simulink model "gm_pwm_fpga_slrt"  (R2020b)
settings: Solver=FixedStepDiscrete  StartTime=0.0  StopTime=5  FixedStep=1e-3  RelTol=1e-3
PostLoadFcn:
  | try
  | cell = struct2cell(dir(fullfile(speedgoatroot_hdlb, 'hdlsrc', 'pwm', '*.vhd')));
  | addSourceFiles = strjoin(fullfile(cell(2,:),cell(1,:)), ';');
  | hdlset_param('pwm_example_hdlc/DUT PWM and CAP', 'IPCoreAdditionalFiles', addSourceFiles);
  | end
undefined symbols (not defined in the file): IO334
libraries: speedgoatlib_hdlCoder_IO3xx x5, pwm_cpulib x1
settings Model: ModifiedByFormat=Speedgoat GmbH  Creator=Speedgoat GmbH  LastModifiedBy=Speedgoat GmbH
settings SolverCC: ConcurrentTasks=on  PositivePriorityOrder=on
settings DataIOCC: LimitDataPoints=on  SaveFormat=Array  ReturnWorkspaceOutputs=off
settings OptimizationCC: BlockReduction=off  ConditionallyExecuteInputs=off  DefaultParameterBehavior=Inlined  OptimizeBlockIOStorage=off
settings DebuggingCC: AlgebraicLoopMsg=error  UnderspecifiedInitializationDetection=Classic  MergeDetectMultiDrivingBlocksExec=none  SolverPrmCheckMsg=warning  SingleTaskRateTransMsg=error  TasksWithSamePriorityMsg=none  PregeneratedLibrarySubsystemCodeDiagnostic=none  SFUnexpectedBacktrackingDiag=warning  SFNoUnconditionalDefaultTransitionDiag=warning  SFExecutionAtInitializationDiag=none  ArithmeticOperatorsInVariantConditions=warning
settings HardwareCC: ProdBitPerLong=64  ProdLongLongMode=on  ProdHWDeviceType=Intel->x86-64 (Linux 64)
settings ModelReferenceCC: PropagateSignalLabelsOutOfModel=off
settings SFSimCC: SimUseLocalCustomCode=off  CustomCodeUndefinedFunction=UseInterfaceOnly
settings RTWCC: Description=Simulink Real-Time  SystemTargetFile=slrealtime.tlc  TemplateMakefile=slrealtime_default_tmf  RTWUseLocalCustomCode=off  Toolchain=Simulink Real-Time Toolchain  BuildConfiguration=Faster Runs  CodeExecutionProfiling=on  TargetLang=C++
settings CodeAppCC: StateflowObjectComments=on
settings ConfigComp: CovMetricSettings=dw  CovSaveCumulativeToWorkspaceVar=on  CovSaveSingleToWorkspaceVar=on  CovExternalEMLEnable=off

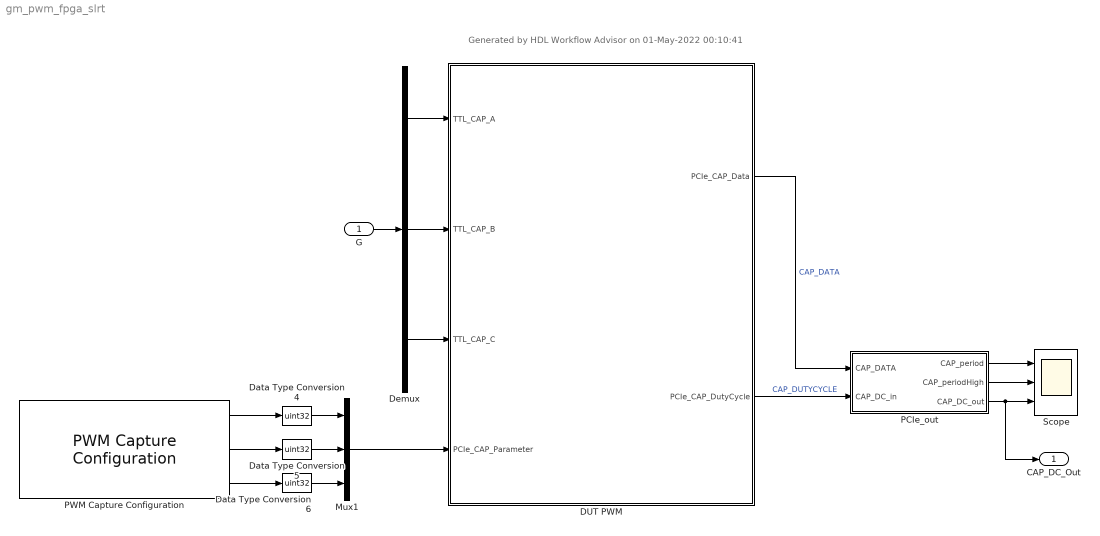
== system gm_pwm_fpga_slrt ==
  note: Generated by HDL Workflow Advisor on 01-May-2022 00:10:41
  G : Inport
  DUT PWM : Subsystem  mask(Speedgoat IO334-325k Interface Block){module_id=1, slot=-1, ts=-1, PullRPort0=pull-up 3.3V, VioPort0=3.3V, PullRPort1=pull-up 3.3V, VioPort1=3.3V, PullRPort2=pull-up 3.3V, VioPort2=3.3V, PullRPort3=pull-up 3.3V, VioPort3=3.3V, PullRPort4=pull-up 3.3V, VioPort4=3.3V, PullRPort5=pull-up 3.3V, VioPort5=3.3V, PullRPort6=pull-up 3.3V, VioPort6=3.3V, FpgaFreq=100}
      mask prompts: module_id "FPGA Module Identifier:"; slot "PCI slot (-1: autosearch):"; ts "Sample time:"; PullRPort0 "pull resistor"; VioPort0 "I/O voltage"; PullRPort1 "pull resistor"; VioPort1 "I/O voltage"; PullRPort2 "pull resistor"; VioPort2 "I/O voltage"; PullRPort3 "pull resistor"; VioPort3 "I/O voltage"; PullRPort4 "pull resistor"; VioPort4 "I/O voltage"; PullRPort5 "pull resistor"; VioPort5 "I/O voltage"; PullRPort6 "pull resistor"; VioPort6 "I/O voltage"; FpgaFreq "FPGA Frequency [MHz]"
      mask help: Simulink Real-Time Interface Block for Speedgoat IO334-325k.
      mask init:
      | hdlslrt.backend.mfpgaparameters;
      mask Help: eval('speedgoatdoc_hdlc')
      mask TypeOptions PullRPort0: Port Settings -2x/PullRPort0
      mask Callback PullRPort0: sg_fpga_HDLCoder_io3xx_2x_m(2)
      mask TypeOptions VioPort0: Port Settings -2x/VioPort0
      mask Callback VioPort0: sg_fpga_HDLCoder_io3xx_2x_m(2)
      mask TypeOptions PullRPort1: Port Settings -2x/PullRPort1
      mask Callback PullRPort1: sg_fpga_HDLCoder_io3xx_2x_m(2)
      mask TypeOptions VioPort1: Port Settings -2x/VioPort1
      mask Callback VioPort1: sg_fpga_HDLCoder_io3xx_2x_m(2)
      mask TypeOptions PullRPort2: Port Settings -2x/PullRPort2
      mask Callback PullRPort2: sg_fpga_HDLCoder_io3xx_2x_m(2)
      mask TypeOptions VioPort2: Port Settings -2x/VioPort2
      mask Callback VioPort2: sg_fpga_HDLCoder_io3xx_2x_m(2)
      mask TypeOptions PullRPort3: Port Settings -2x/PullRPort3
      mask Callback PullRPort3: sg_fpga_HDLCoder_io3xx_2x_m(2)
      mask TypeOptions VioPort3: Port Settings -2x/VioPort3
      mask Callback VioPort3: sg_fpga_HDLCoder_io3xx_2x_m(2)
      mask TypeOptions PullRPort4: Port Settings -2x/PullRPort4
      mask Callback PullRPort4: sg_fpga_HDLCoder_io3xx_2x_m(2)
      mask TypeOptions VioPort4: Port Settings -2x/VioPort4
      mask Callback VioPort4: sg_fpga_HDLCoder_io3xx_2x_m(2)
      mask TypeOptions PullRPort5: Port Settings -2x/PullRPort5
      mask Callback PullRPort5: sg_fpga_HDLCoder_io3xx_2x_m(2)
      mask TypeOptions VioPort5: Port Settings -2x/VioPort5
      mask Callback VioPort5: sg_fpga_HDLCoder_io3xx_2x_m(2)
      mask TypeOptions PullRPort6: Port Settings -2x/PullRPort6
      mask Callback PullRPort6: sg_fpga_HDLCoder_io3xx_2x_m(2)
      mask TypeOptions VioPort6: Port Settings -2x/VioPort6
      mask Callback VioPort6: sg_fpga_HDLCoder_io3xx_2x_m(2)
      mask DialogControl IO33421 Prompt: IO334-21
      mask DialogControl port1 Prompt: Port 1
      mask DialogControl port2 Prompt: Port 2
      mask DialogControl port3 Prompt: Port 3
      mask DialogControl port4 Prompt: Port 4
      mask DialogControl port5 Prompt: Port 5
      mask DialogControl port6 Prompt: Port 6
      mask DialogControl port7 Prompt: Port 7
      mask Display:
      | SetupBlkPath = find_system(gcb, 'LookUnderMasks', 'all', 'FollowLinks', 'on', 'regexp', 'on', 'Name', 'IO3(\d|x){2}\s+Setup' );
      | SetupBlkPath = SetupBlkPath{1};
      | TS = get_param(SetupBlkPath,'timestamp_mcs');
      | disp(sprintf('Speedgoat IO334-325k\nFPGA I/O Module\n\nTimestamp\n%s\n\nReference Design\nVersion 2.1\n\nMatlab R2020b\n\nPCIe Link Width: X4\nRear Plugin: -21\nAurora Mode: None\nAurora Byteswap: true\n', TS))
  Data Type Conversion4 : DataTypeConversion  OutDataTypeStr=uint32
  Data Type Conversion5 : DataTypeConversion  OutDataTypeStr=uint32
  Data Type Conversion6 : DataTypeConversion  OutDataTypeStr=uint32
  Demux : Demux  Outputs=3
  Mux1 : Mux  Inputs=3
  PCIe_out : Subsystem
  PWM Capture Configuration : pwm_cpulib/PWM Capture Configuration  FPGA_freq=100e6  n_channels=1  captureMode=High transitions triggered  captureTimeout=0  PWM_pattern_en=off
      settings: SourceProductName=Simulink Real-Time: Speedgoat HDL Blockset
  Scope : Scope  NumInputPorts=3
  CAP_DC_Out : Outport  VectorParamsAs1DForOutWhenUnconnected=off
  wires:
  Mux1/1 -> DUT PWM/4(PCIe_CAP_Parameter)
  Data Type Conversion6/1 -> Mux1/3
  Data Type Conversion5/1 -> Mux1/2
  Data Type Conversion4/1 -> Mux1/1
  PWM Capture Configuration/2 -> Data Type Conversion5/1
  PWM Capture Configuration/3 -> Data Type Conversion6/1
  PWM Capture Configuration/1 -> Data Type Conversion4/1
  PCIe_out/1(CAP_period) -> Scope/1
  PCIe_out/2(CAP_periodHigh) -> Scope/2
  PCIe_out/3(CAP_DC_out) -> CAP_DC_Out/1, Scope/3
  DUT PWM/1(PCIe_CAP_Data) -> PCIe_out/1(CAP_DATA)  "CAP_DATA"
  DUT PWM/2(PCIe_CAP_DutyCycle) -> PCIe_out/2(CAP_DC_in)  "CAP_DUTYCYCLE"
  G/1 -> Demux/1
  Demux/1 -> DUT PWM/1(TTL_CAP_A)
  Demux/2 -> DUT PWM/2(TTL_CAP_B)
  Demux/3 -> DUT PWM/3(TTL_CAP_C)

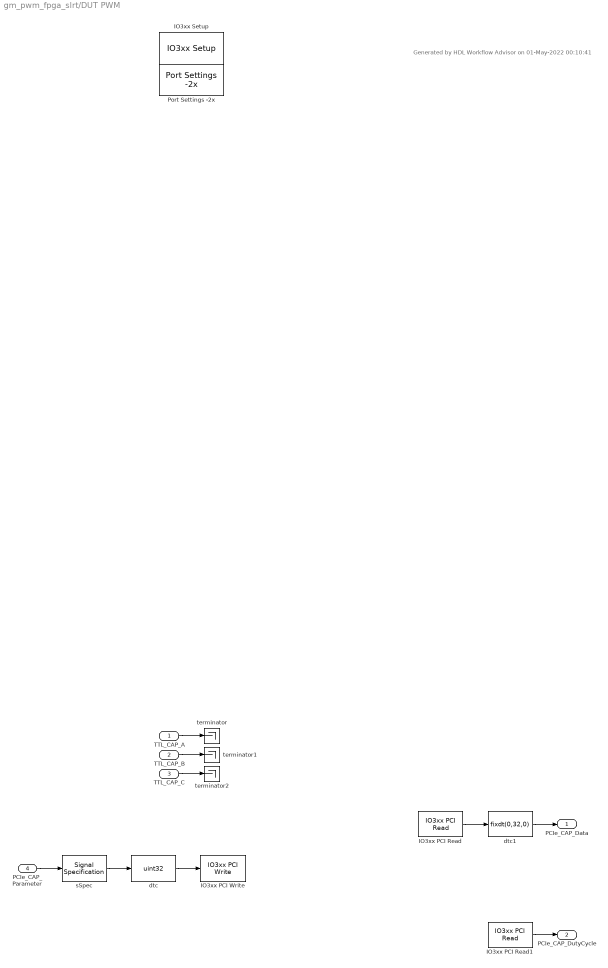
== system gm_pwm_fpga_slrt/DUT PWM ==
  note: Generated by HDL Workflow Advisor on 01-May-2022 00:10:41
  TTL_CAP_A : Inport
  TTL_CAP_B : Inport  Port=2
  TTL_CAP_C : Inport  Port=3
  PCIe_CAP_Parameter : Inport  Port=4
  IO3xx PCI Read : speedgoatlib_hdlCoder_IO3xx/IO3xx PCI Read  device_id=1  module_id=module_id  board_type=IO334-325k  port_name=PCIe_CAP_Data  port_offset=hex2dec('180')  port_type=uint32  port_dim=18  strobe=hex2dec('200')  sample_time=ts
  IO3xx PCI Read1 : speedgoatlib_hdlCoder_IO3xx/IO3xx PCI Read  device_id=1  module_id=module_id  board_type=IO334-325k  port_name=PCIe_CAP_DutyCycle  port_offset=hex2dec('120')  port_type=single  port_dim=3  strobe=hex2dec('130')  sample_time=ts
  IO3xx PCI Write : speedgoatlib_hdlCoder_IO3xx/IO3xx PCI Write  device_id=1  module_id=module_id  board_type=IO334-325k  port_name=PCIe_CAP_Parameter  port_offset=hex2dec('100')  port_type=uint32  port_dim=3  strobe=hex2dec('110')  sample_time=ts
  IO3xx Setup : speedgoatlib_hdlCoder_IO3xx/IO3xx Setup  mdl_ss_name=pwm_fpga/DUT PWM  board_type=IO334-325k  fpga_sync_mode=on  reset_mode=on  device_id=1  module_id=module_id  pci_slot=slot  fpga_mat_file=hdl_prj\hdlsrc\pwm_fpga\DUTPWM.mat  timestamp_mcs=05/01/22 00:05:42  timestamp=2204302246  tsreg=hex2dec('8')  bsf_file=DUTPWM_2204302246.mcs  mcs=0
  Port Settings -2x : speedgoatlib_hdlCoder_IO3xx/Port Settings -2x  module_id=module_id  rearIO=-21  PullRPort0=pull-up 3.3V  VioPort0=3.3V  PullRPort1=pull-up 3.3V  VioPort1=3.3V  PullRPort2=pull-up 3.3V  VioPort2=3.3V  PullRPort3=pull-up 3.3V  VioPort3=3.3V  PullRPort4=pull-up 3.3V  VioPort4=3.3V  PullRPort5=pull-up 3.3V  VioPort5=3.3V  PullRPort6=pull-up 3.3V  VioPort6=3.3V
  dtc : DataTypeConversion  OutDataTypeStr=uint32  ConvertRealWorld=Stored Integer (SI)  RndMeth=Zero
  dtc1 : DataTypeConversion  OutDataTypeStr=fixdt(0,32,0)  ConvertRealWorld=Stored Integer (SI)  RndMeth=Zero
  sSpec : SignalSpecification  OutDataTypeStr=fixdt(0,32,0)
  terminator : Terminator
  terminator1 : Terminator
  terminator2 : Terminator
  PCIe_CAP_Data : Outport  VectorParamsAs1DForOutWhenUnconnected=off
  PCIe_CAP_DutyCycle : Outport  Port=2  VectorParamsAs1DForOutWhenUnconnected=off
  wires:
  TTL_CAP_A/1 -> terminator/1
  TTL_CAP_B/1 -> terminator1/1
  TTL_CAP_C/1 -> terminator2/1
  PCIe_CAP_Parameter/1 -> sSpec/1
  sSpec/1 -> dtc/1
  dtc/1 -> IO3xx PCI Write/1
  dtc1/1 -> PCIe_CAP_Data/1
  IO3xx PCI Read/1 -> dtc1/1
  IO3xx PCI Read1/1 -> PCIe_CAP_DutyCycle/1

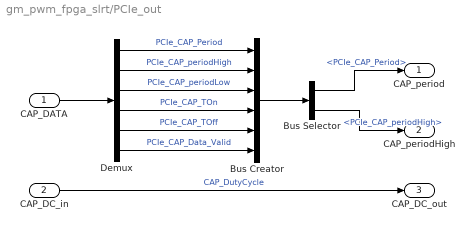
== system gm_pwm_fpga_slrt/PCIe_out ==
  CAP_DATA : Inport
  CAP_DC_in : Inport  Port=2
  Bus Creator : BusCreator  Inputs=6
  Bus Selector : BusSelector  OutputSignals=PCIe_CAP_Period,PCIe_CAP_periodHigh
  Demux : Demux  Outputs=6
  CAP_period : Outport
  CAP_periodHigh : Outport  Port=2
  CAP_DC_out : Outport  Port=3
  wires:
  CAP_DATA/1 -> Demux/1
  Demux/5 -> Bus Creator/5  "PCIe_CAP_TOff"
  Demux/1 -> Bus Creator/1  "PCIe_CAP_Period"
  Bus Creator/1 -> Bus Selector/1
  Demux/4 -> Bus Creator/4  "PCIe_CAP_TOn"
  Demux/2 -> Bus Creator/2  "PCIe_CAP_periodHigh"
  Demux/3 -> Bus Creator/3  "PCIe_CAP_periodLow"
  Demux/6 -> Bus Creator/6  "PCIe_CAP_Data_Valid"
  Bus Selector/1 -> CAP_period/1  "<PCIe_CAP_Period>"
  Bus Selector/2 -> CAP_periodHigh/1  "<PCIe_CAP_periodHigh>"
  CAP_DC_in/1 -> CAP_DC_out/1  "CAP_DutyCycle"
